simulink model "untitled123"  (R2021a)
settings: Solver=FixedStepDiscrete  StartTime=0.0  StopTime=1.0  RelTol=1e-3
libraries: simulink x2, SignalEditorBlockLib x2
settings Model: Creator=voval  LastModifiedBy=voval
settings OptimizationCC: DefaultParameterBehavior=Inlined  EnhancedBackFolding=on  PassReuseOutputArgsAs=Individual arguments  ZeroExternalMemoryAtStartup=off  ZeroInternalMemoryAtStartup=off  OptimizeBlockOrder=speed  DifferentSizesBufferReuse=on  OptimizationCustomize=off  EfficientTunableParamExpr=on
settings DebuggingCC: ParameterTunabilityLossMsg=error
settings HardwareCC: ProdBitPerInt=16  ProdBitPerPointer=16  ProdBitPerSizeT=16  ProdBitPerPtrDiffT=16  ProdLargestAtomicFloat=None  ProdWordSize=16  ProdHWDeviceType=Atmel->AVR (8-bit)
settings SFSimCC: MATLABDynamicMemAlloc=off
settings RTWCC: SystemTargetFile=ert.tlc  TemplateMakefile=ert_default_tmf  GenerateReport=on  LaunchReport=on
settings CodeAppCC: ForceParamTrailComments=on  IgnoreCustomStorageClasses=off  OperatorAnnotations=on  SimulinkDataObjDesc=on  SFDataObjDesc=on  InsertBlockDesc=on
settings ERTTargetCC: TargetLangStandard=C99 (ISO)  GenerateSampleERTMain=on  InlinedParameterPlacement=NonHierarchical  ERTCustomFileTemplate=example_file_process.tlc  ERTFilePackagingFormat=Compact

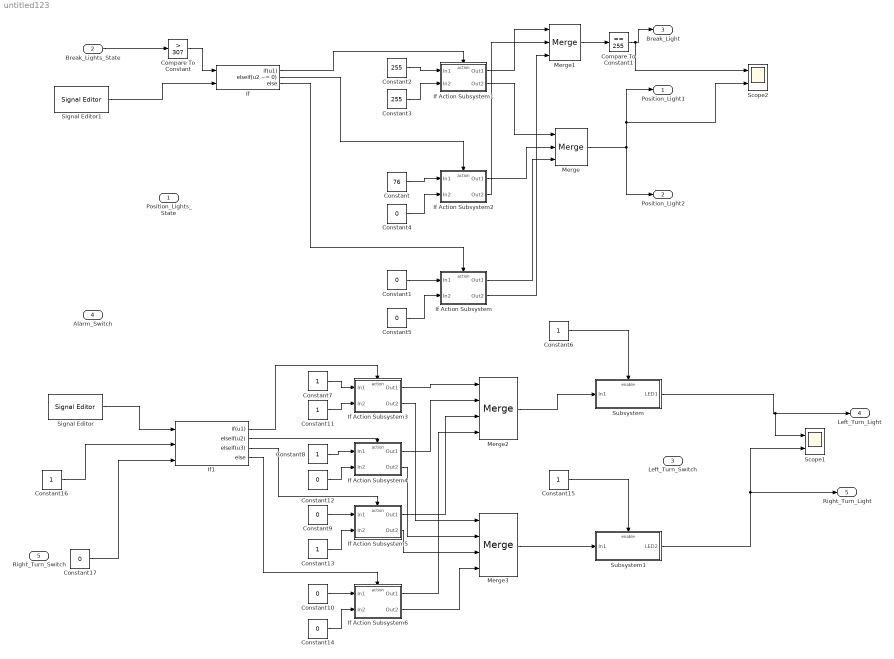
== system untitled123 ==
  Position_Lights_State : Inport  OutDataTypeStr=boolean
  Break_Lights_State : Inport  Port=2  OutDataTypeStr=uint16
  Left_Turn_Switch : Inport  Port=3  OutDataTypeStr=boolean
  Alarm_Switch : Inport  Port=4  OutDataTypeStr=boolean
  Right_Turn_Switch : Inport  Port=5  OutDataTypeStr=boolean
  Compare To Constant : simulink/Logic and Bit Operations/Compare To Constant  relop=>  const=307  OutDataTypeStr=boolean
  Compare To Constant1 : simulink/Logic and Bit Operations/Compare To Constant  relop===  const=255  OutDataTypeStr=boolean
  Constant : Constant  Value=76  OutDataTypeStr=uint8
  Constant1 : Constant  Value=0  OutDataTypeStr=uint8
  Constant{9..10,12,14,17} (5 alike) : Constant  Value=0  OutDataTypeStr=boolean
  Constant{6..8,11,13,15..16} (7 alike) : Constant  OutDataTypeStr=boolean
  Constant2 : Constant  Value=255  OutDataTypeStr=uint8
  Constant3 : Constant  Value=255  OutDataTypeStr=uint8
  Constant4 : Constant  Value=0  OutDataTypeStr=uint8
  Constant5 : Constant  Value=0  OutDataTypeStr=uint8
  If : If  NumInputs=2  IfExpression=u1  ElseIfExpressions=u2 ~= 0
  If Action Subsystem : Subsystem  TreatAsAtomicUnit=on
  If Action Subsystem1 : Subsystem  TreatAsAtomicUnit=on
  If Action Subsystem2 : Subsystem  TreatAsAtomicUnit=on
  If Action Subsystem3 : Subsystem  TreatAsAtomicUnit=on
  If Action Subsystem4 : Subsystem  TreatAsAtomicUnit=on
  If Action Subsystem5 : Subsystem  TreatAsAtomicUnit=on
  If Action Subsystem6 : Subsystem  TreatAsAtomicUnit=on
  If1 : If  NumInputs=3  IfExpression=u1  ElseIfExpressions=u2, u3
  Merge : Merge  Inputs=3
  Merge1 : Merge  Inputs=3
  Merge2 : Merge  Inputs=4
  Merge3 : Merge  Inputs=4
  Scope1 : Scope  NumInputPorts=2
  Scope2 : Scope  NumInputPorts=2
  Signal Editor : SignalEditorBlockLib/Signal Editor  FileName=SceneryOnAlarm.mat  ActiveScenario=Scenario  ActiveSignal=Signal 1  IsBus=off  OutputBusObjectStr=Bus: BusObject  SampleTime=0  Interpolate=off  ZeroCross=off  OutputAfterFinalValue=Setting to zero  Unit=inherit  PreserveSignalName=on
  Signal Editor1 : SignalEditorBlockLib/Signal Editor  FileName=SceneryOnPostitionLights.mat  ActiveScenario=Scenario  ActiveSignal=Signal 1  IsBus=off  OutputBusObjectStr=Bus: BusObject  SampleTime=0  Interpolate=off  ZeroCross=off  OutputAfterFinalValue=Setting to zero  Unit=inherit  PreserveSignalName=on
  Subsystem : Subsystem
  Subsystem1 : Subsystem
  Position_Light1 : Outport  OutDataTypeStr=uint8
  Position_Light2 : Outport  Port=2  OutDataTypeStr=uint8
  Break_Light : Outport  Port=3  OutDataTypeStr=boolean
  Left_Turn_Light : Outport  Port=4  OutDataTypeStr=boolean
  Right_Turn_Light : Outport  Port=5  OutDataTypeStr=boolean
  wires:
  Constant/1 -> If Action Subsystem2/1(In1)
  Signal Editor1/1 -> If/2
  If/3 -> If Action Subsystem/Action
  Constant1/1 -> If Action Subsystem/1(In1)
  If/1 -> If Action Subsystem1/Action
  If/2 -> If Action Subsystem2/Action
  Merge/1 -> Scope2/2, Position_Light1/1, Position_Light2/1
  If Action Subsystem/1(Out1) -> Merge/3
  If Action Subsystem2/1(Out1) -> Merge/2
  Break_Lights_State/1 -> Compare To Constant/1
  Compare To Constant/1 -> If/1
  Constant4/1 -> If Action Subsystem2/2(In2)
  Constant5/1 -> If Action Subsystem/2(In2)
  If Action Subsystem2/2(Out2) -> Merge1/2
  If Action Subsystem/2(Out2) -> Merge1/3
  Constant3/1 -> If Action Subsystem1/2(In2)
  Constant2/1 -> If Action Subsystem1/1(In1)
  If Action Subsystem1/1(Out1) -> Merge1/1
  If Action Subsystem1/2(Out2) -> Merge/1
  Constant6/1 -> Subsystem/Enable
  Constant16/1 -> If1/2
  Constant17/1 -> If1/3
  Signal Editor/1 -> If1/1
  If1/1 -> If Action Subsystem3/Action
  If1/2 -> If Action Subsystem4/Action
  Constant9/1 -> If Action Subsystem5/1(In1)
  Constant7/1 -> If Action Subsystem3/1(In1)
  Constant11/1 -> If Action Subsystem3/2(In2)
  Constant8/1 -> If Action Subsystem4/1(In1)
  Constant12/1 -> If Action Subsystem4/2(In2)
  If1/3 -> If Action Subsystem5/Action
  Constant13/1 -> If Action Subsystem5/2(In2)
  If1/4 -> If Action Subsystem6/Action
  Constant10/1 -> If Action Subsystem6/1(In1)
  Constant14/1 -> If Action Subsystem6/2(In2)
  If Action Subsystem3/1(Out1) -> Merge2/1
  If Action Subsystem4/1(Out1) -> Merge2/2
  If Action Subsystem5/1(Out1) -> Merge2/3
  If Action Subsystem6/1(Out1) -> Merge2/4
  Merge2/1 -> Subsystem/1(In1)
  Constant15/1 -> Subsystem1/Enable
  If Action Subsystem3/2(Out2) -> Merge3/1
  If Action Subsystem4/2(Out2) -> Merge3/2
  If Action Subsystem5/2(Out2) -> Merge3/3
  If Action Subsystem6/2(Out2) -> Merge3/4
  Merge3/1 -> Subsystem1/1(In1)
  Subsystem/1(LED1) -> Scope1/1, Left_Turn_Light/1
  Merge1/1 -> Compare To Constant1/1
  Compare To Constant1/1 -> Scope2/1, Break_Light/1
  Subsystem1/1(LED2) -> Scope1/2, Right_Turn_Light/1

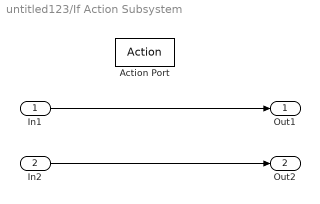
== system untitled123/If Action Subsystem ==
  In1 : Inport  OutDataTypeStr=uint8
  In2 : Inport  Port=2  OutDataTypeStr=uint8
  Action Port : ActionPort  ActionPortLabel=else
  Out1 : Outport  OutDataTypeStr=uint8
  Out2 : Outport  Port=2  OutDataTypeStr=uint8
  wires:
  In1/1 -> Out1/1
  In2/1 -> Out2/1

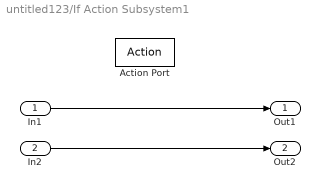
== system untitled123/If Action Subsystem1 ==
  In1 : Inport  OutDataTypeStr=uint8
  In2 : Inport  Port=2  OutDataTypeStr=uint8
  Action Port : ActionPort  ActionPortLabel=if(u1)
  Out1 : Outport  OutDataTypeStr=uint8
  Out2 : Outport  Port=2  OutDataTypeStr=uint8
  wires:
  In1/1 -> Out1/1
  In2/1 -> Out2/1

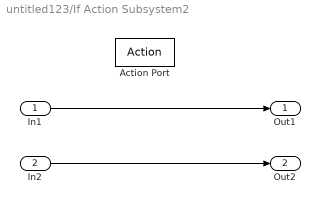
== system untitled123/If Action Subsystem2 ==
  In1 : Inport  OutDataTypeStr=uint8
  In2 : Inport  Port=2  OutDataTypeStr=uint8
  Action Port : ActionPort  ActionPortLabel=elseif(u2 ~= 0)
  Out1 : Outport  OutDataTypeStr=uint8
  Out2 : Outport  Port=2  OutDataTypeStr=uint8
  wires:
  In1/1 -> Out1/1
  In2/1 -> Out2/1

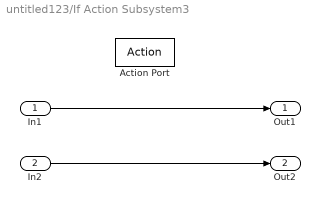
== system untitled123/If Action Subsystem3 ==
  In1 : Inport  OutDataTypeStr=boolean
  In2 : Inport  Port=2  OutDataTypeStr=boolean
  Action Port : ActionPort  ActionPortLabel=if(u1)
  Out1 : Outport  OutDataTypeStr=boolean
  Out2 : Outport  Port=2  OutDataTypeStr=boolean
  wires:
  In1/1 -> Out1/1
  In2/1 -> Out2/1

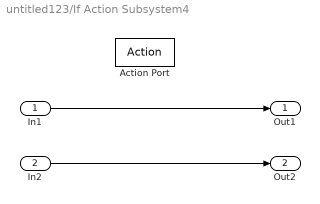
== system untitled123/If Action Subsystem4 ==
  In1 : Inport  OutDataTypeStr=boolean
  In2 : Inport  Port=2  OutDataTypeStr=boolean
  Action Port : ActionPort  ActionPortLabel=elseif(u2)
  Out1 : Outport  OutDataTypeStr=boolean
  Out2 : Outport  Port=2  OutDataTypeStr=boolean
  wires:
  In1/1 -> Out1/1
  In2/1 -> Out2/1

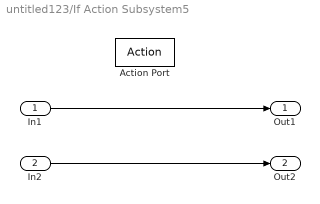
== system untitled123/If Action Subsystem5 ==
  In1 : Inport  OutDataTypeStr=boolean
  In2 : Inport  Port=2  OutDataTypeStr=boolean
  Action Port : ActionPort  ActionPortLabel=elseif( u3)
  Out1 : Outport  OutDataTypeStr=boolean
  Out2 : Outport  Port=2  OutDataTypeStr=boolean
  wires:
  In1/1 -> Out1/1
  In2/1 -> Out2/1

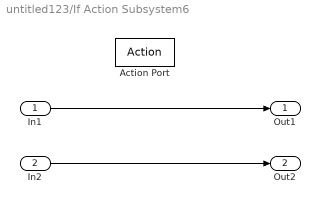
== system untitled123/If Action Subsystem6 ==
  In1 : Inport  OutDataTypeStr=boolean
  In2 : Inport  Port=2  OutDataTypeStr=boolean
  Action Port : ActionPort  ActionPortLabel=else
  Out1 : Outport  OutDataTypeStr=boolean
  Out2 : Outport  Port=2  OutDataTypeStr=boolean
  wires:
  In1/1 -> Out1/1
  In2/1 -> Out2/1

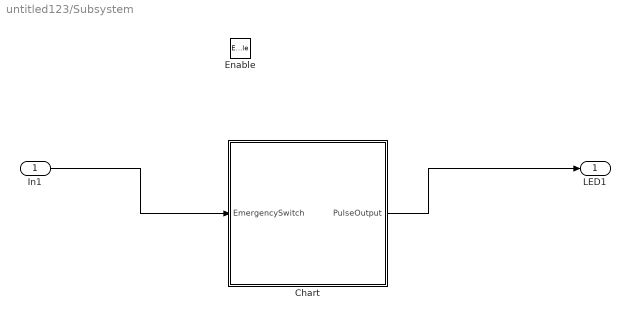
== system untitled123/Subsystem ==
  In1 : Inport  OutDataTypeStr=boolean
  Enable : EnablePort
  Chart : Stateflow chart  TreatAsAtomicUnit=on
  LED1 : Outport  OutDataTypeStr=boolean
  wires:
  In1/1 -> Chart/1(EmergencySwitch)
  Chart/1(PulseOutput) -> LED1/1

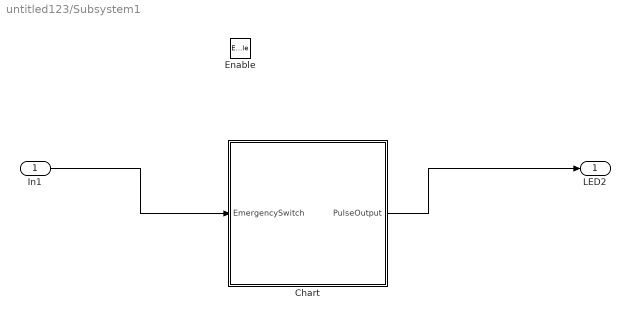
== system untitled123/Subsystem1 ==
  In1 : Inport  OutDataTypeStr=boolean
  Enable : EnablePort
  Chart : Stateflow chart  TreatAsAtomicUnit=on
  LED2 : Outport  OutDataTypeStr=boolean
  wires:
  In1/1 -> Chart/1(EmergencySwitch)
  Chart/1(PulseOutput) -> LED2/1

== stateflow chart untitled123/Subsystem1/Chart ==
  state StateHigh
    en: PulseOutput = false;
  state StateLow
    en: PulseOutput = true;
  (default) -> StateHigh
  StateHigh -> StateLow : [EmergencySwitch && after(5,tick)]
  StateLow -> StateHigh : [after(5,tick)]
  data: EmergencySwitch input boolean; PulseOutput output boolean

== stateflow chart untitled123/Subsystem/Chart ==
  state StateHigh
    en: PulseOutput = false;
  state StateLow
    en: PulseOutput = true;
  (default) -> StateHigh
  StateHigh -> StateLow : [EmergencySwitch && after(5, tick)]
  StateLow -> StateHigh : [after(5,tick)]
  data: EmergencySwitch input; PulseOutput output
